simulink model "calibrazione_M"  (Simulink 7.7)
settings: Solver=ode45  StartTime=0.0  StopTime=10  RelTol=1e-3
undefined symbols (not defined in the file or in its folder): aerosimlib, Earth, WMM
libraries: aerolibgravity2 x1
settings Model: Creator=andrea  LastModifiedBy=Fede
settings OptimizationCC: InitFltsAndDblsToZero=on  OptimizeModelRefInitCode=on  LifeSpan=1
settings DebuggingCC: StrictBusMsg=Warning
settings SFSimCC: SimParseCustomCode=off
settings RTWCC: SystemTargetFile=ert.tlc  TemplateMakefile=ert_default_tmf  Description=Embedded Coder  ProcessScript=ert_make_rtw_hook
settings CodeAppCC: IgnoreCustomStorageClasses=off
settings ERTTargetCC: FunctionExecutionProfile=off  MultiwordLength=2048  GenerateSampleERTMain=on  ERTCustomFileTemplate=example_file_process.tlc  ConvertIfToSwitch=off

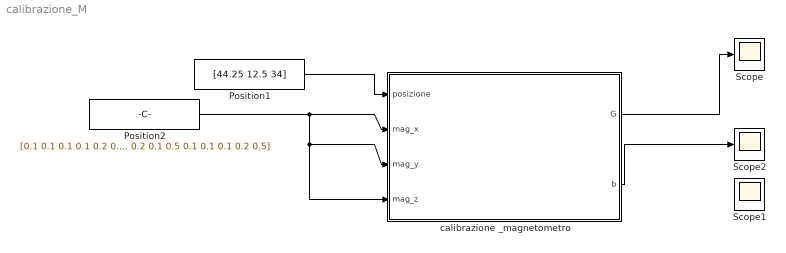
== system calibrazione_M ==
  Position1 : Constant  Value=[44.25 12.5 34]
  Position2 : Constant  Value=[0.1 0.1 0.1 0.1 0.2 0.1 0.5 0.1 0.1 0.1 0.2 0.5 0.1 0.1 0.1 0.1 0.2 0.1 0.5 0.1 0.1 0.1 0.2 0.5 0.1 0.1 0.1 0.1 0.2 0.1 0.5 0.1 0.1 0.1 0.2 0.5 0.1 0.1 0.1 0.1 0.2 0.1 0.5 0.1 0.1 0.1 0.2 0.5 0.1 0.1 0.1 0.1 0.2 0.1 0.5 0.1 0.1 0.1 0.2 0.5 0.1 0.1 0.1 0.1 0.2 0.1 0.5 0.1 0.1 0.1 0.2 0.5 0.1 0.1 0.1 0.1 0.2 0.1 0.5 0.1 0.1 0.1 0.2 0.5 0.1 0.1 0.1 0.1 0.2 0.1 0.5 0.1 0.1 0.1 0.2 0.5 0.1 0.1 0.1 0.1 0.2 0.1 0.5 0.1 0.1 0.1 0.2 0.5 0.1 0.1 0.1 0.1 0.2 0.1 0.5 0.1 0.1 0.1 0.2 0.5 0.1 0.1 0.1 0.1 0.2 0.1 0.5 0.1 0.1 0.1 0.2 0.5 0.1 0.1 0.1 0.1 0.2 0.1 0.5 0.1 0.1 0.1 0.2 0.5 0.1 0.1 0.1 0.1 0.2 0.1 0.5 0.1 0.1 0.1 0.2 0.5 0.1 0.1 0.1 0.1 0.2 0.1 0.5 0.1 0.1 0.1 0.2 0.5]
  Scope : Scope
  Scope1 : Scope
  Scope2 : Scope
      settings: SaveName=ScopeData2
  calibrazione _magnetometro : Subsystem
  wires:
  Position1/1 -> calibrazione _magnetometro/1(posizione)
  calibrazione _magnetometro/1(G) -> Scope/1
  calibrazione _magnetometro/2(b) -> Scope2/1
  ? -> Scope1/1
  Position2/1 -> calibrazione _magnetometro/2(mag_x), calibrazione _magnetometro/3(mag_y), calibrazione _magnetometro/4(mag_z)

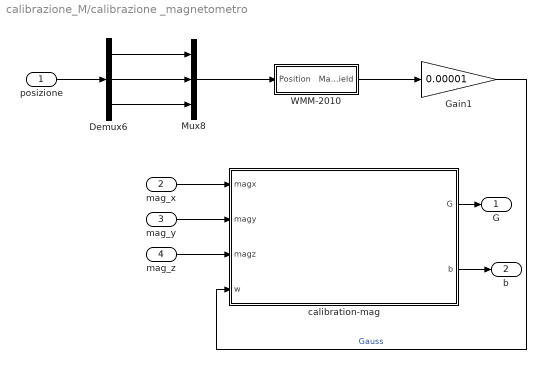
== system calibrazione_M/calibrazione _magnetometro ==
  posizione : Inport
  mag_x : Inport  Port=2
  mag_y : Inport  Port=3
  mag_z : Inport  Port=4
  Demux6 : Demux  Outputs=3
  Gain1 : Gain  Gain=0.00001
  Mux8 : Mux  Inputs=3
  WMM-2010 : Subsystem  AncestorBlock=aerosimlib/Earth/WMM-2000  mask(WMM-2000){wmmfile='C:\\Programmmi\\AeroSim\\wmm.cof', simdate=[26 05 2011]}
      mask prompts: wmmfile "WMM coefficient file:"; simdate "Simulation date [Day Month Year]:"
      mask help: The World Magnetic Model returns the Earth magnetic field components in body axes at current aircraft location.
      mask Help:
      | The block provides the magnetic field components at current aircraft location.
      | <P><B>Inputs:</B>
      | <LI>Position = the 3x1 vector of aircraft location [Latitude Longitude Altitude] in [rad rad m]</LI>
      | <LI>DCM = the frame transformation matrix from navigation to body frame</LI>
      | </P>
      | <P><B>Output:</B>
      | <LI>MagField = the 3x1 vector of magnetic field components in body axes</LI>
      | </P>
      | <P><B>Parameters:</B>
      | <LI>WMM coefficient file = the path to the WMM coefficient file, as a 'string'</LI>
      | <LI>Simulation date = the 1x3 vector of current date [Day Month Year]</LI>
      | </P>
  calibration-mag : Stateflow chart  TreatAsAtomicUnit=on
  G : Outport
  b : Outport  Port=2
  wires:
  Demux6/2 -> Mux8/2
  Demux6/1 -> Mux8/1
  Demux6/3 -> Mux8/3
  posizione/1 -> Demux6/1
  WMM-2010/1(MagField) -> Gain1/1
  Mux8/1 -> WMM-2010/1(Position)
  mag_x/1 -> calibration-mag/1(magx)
  mag_y/1 -> calibration-mag/2(magy)
  calibration-mag/1(G) -> G/1
  mag_z/1 -> calibration-mag/3(magz)
  calibration-mag/2(b) -> b/1
  Gain1/1 -> calibration-mag/4(w)  "Gauss"

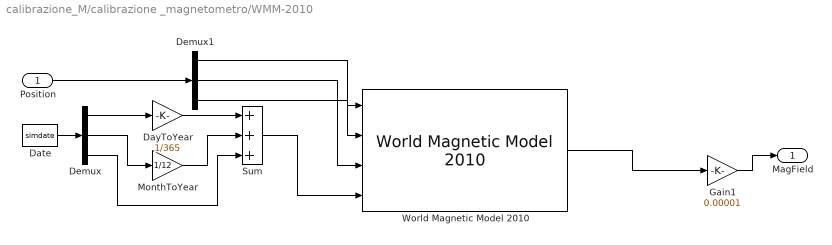
== system calibrazione_M/calibrazione _magnetometro/WMM-2010 ==
  Position : Inport  OutDataTypeStr=double  PortDimensions=[3 1]
  Date : Constant  Value=simdate
  DayToYear : Gain  Gain=1/365  SaturateOnIntegerOverflow=on  OutDataTypeStr=Inherit: Same as input  ParamDataTypeStr=Inherit: Same as input
  Demux : Demux  Outputs=3
  Demux1 : Demux  Outputs=3
  Gain1 : Gain  Gain=0.00001
  MonthToYear : Gain  Gain=1/12  SaturateOnIntegerOverflow=on  OutDataTypeStr=Inherit: Same as input  ParamDataTypeStr=Inherit: Same as input
  Sum : Sum  Inputs=+++  SaturateOnIntegerOverflow=on  InputSameDT=on  OutDataTypeStr=Inherit: Same as first input
  World Magnetic Model 2010 : aerolibgravity2/World Magnetic Model 2010  SystemSampleTime=-1  units=Metric (MKS)  time_in=on  month=January  day=1  year=2010  action=Error  h_out=off  dec_out=off  inc_out=off  ti_out=off
  MagField : Outport
  wires:
  Sum/1 -> World Magnetic Model 2010/4
  MonthToYear/1 -> Sum/2
  Demux/3 -> Sum/3
  Demux/2 -> MonthToYear/1
  DayToYear/1 -> Sum/1
  Demux/1 -> DayToYear/1
  Date/1 -> Demux/1
  Position/1 -> Demux1/1
  Demux1/1 -> World Magnetic Model 2010/2
  Demux1/2 -> World Magnetic Model 2010/3
  Demux1/3 -> World Magnetic Model 2010/1
  Gain1/1 -> MagField/1
  World Magnetic Model 2010/1 -> Gain1/1

== matlab function calibrazione _magnetometro/calibration-mag ==
  data: magx input double; G output double; magy input double; magz input double; w input double; b output double
function [G,b] = fcn(magx, magy,magz,w)
%#codegen
n=40;
%H=[];
H=zeros(n,10);
Hb=zeros(n,3);
B=zeros(n,3);
G=zeros(3,3);
%f=[0:1000:1];
%j=[0:1000:1];
%k=[0:1000:1];
%B=[];
%G=[];
%Hb=[];
h=w(1,:);
hx=magx;
hy=magy;
hz=magz;
for i=1:1:10    %per far si che H abbia almeno 10 elemnti così m>n
    H(i,1)=hx(i)^2;
    H(i,2)=2*hx(i)*hy(i);
    H(i,3)=2*hx(i)*hz(i);
    H(i,4)=hy(i)^2;
    H(i,5)=2*hy(i)*hz(i);
    H(i,6)=hz(i)^2;
    H(i,7)=hx(i);
    H(i,8)=hy(i);
    H(i,9)=hz(i);
    H(i,10)=1;
    Hb(i,1)=hx(i);
    Hb(i,2)=hy(i);
    Hb(i,3)=hz(i);
end
%for i=11:1:length(magx)-1 %ora inizia l'algoritmo
for i=11:1:n -1 %ora inizia l'algoritmo

    H(i,1)=hx(i)^2;
    H(i,2)=2*hx(i)*hy(i);
    H(i,3)=2*hx(i)*hz(i);
    H(i,4)=hy(i)^2;
    H(i,5)=2*hy(i)*hz(i);
    H(i,6)=hz(i)^2;
    H(i,7)=hx(i);
    H(i,8)=hy(i);
    H(i,9)=hz(i);
    H(i,10)=1;
    HH=H'*H; % uso la notazione dell'articolo e creo HH
    [K,P,L]=svd(HH); %HH è una matrice quadrata da cui k è uguale a L
    gsi_norm=K(:,10); % mi fido dell'articolo e prendo la decima colonna che in effetti è relativa al 10° valore singolare che è il + piccolo
    g1=gsi_norm(1);
    g2=gsi_norm(2);
    g3=gsi_norm(3);
    g4=gsi_norm(4);
    g5=gsi_norm(5);
    g6=gsi_norm(6);
    g7=gsi_norm(7);
    g8=gsi_norm(8);
    g9=gsi_norm(9);
    g10=gsi_norm(10);
    gamma=[g1 g2 g3;g2 g4 g5;g3 g5 g6];
    b=-0.5*inv(gamma)*[g7;g8;g9];
    bx=b(1);
    by=b(2);
    bz=b(3);
    B(i,1)=bx; %creo B per notare una convergenza
    B(i,2)=by;
    B(i,3)=bz;
    gsi_modulo=h*h'*(g1*bx^2+2*g2*bx*by+2*g3*bx*bz+g4*by^2+2*g5*by*bz+2*g6*bz^2-g10)^-1; % credo di poter elevare alla -1 tanto è uno scalare
    gsi=gsi_norm*gsi_modulo;
    g1=gsi(1);
    g2=gsi(2);
    g3=gsi(3);
    g4=gsi(4);
    g5=gsi(5);
    g6=gsi(6);
    g7=gsi(7);
    g8=gsi(8);
    g9=gsi(9);
    g10=gsi(10);
    gamma=[g1 g2 g3;g2 g4 g5;g3 g5 g6];
    [U,A,V]=svd(gamma); %per come è costruita gamma è quadrata e simmetrica da cui U è uguale a V
    G=V*sqrt(A)*V';
    b=[bx;by;bz];
    hm=[hx(i);hy(i);hz(i)];
    hb=G*(hm-b);
    Hb(i,1)=hb(1);
    Hb(i,2)=hb(2);
    Hb(i,3)=hb(3);
    %f(i)=norm(hm); %norma del vettore misurato
    %j(i)=norm(hb); %norma del vettore calibrato
    %k(i)=norm(h);  %norma del vettore reale
   
end
